simulink model "adcs_guidance"  (R2024b)
settings: Solver=VariableStepAuto  StartTime=0.0  StopTime=10.0  RelTol=1e-3
undefined symbols (not defined in the file): omega_thresh_high, omega_thresh_low
settings Model: DataDictionary=adcs_params.sldd  Creator=natha  LastModifiedBy=natha

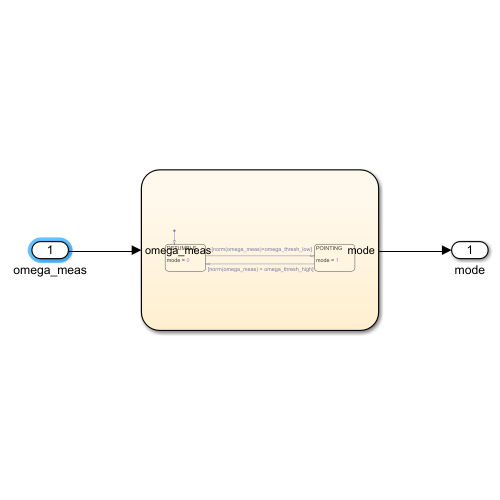
[thumbnail: Simulink's stored preview of the top-level diagram]
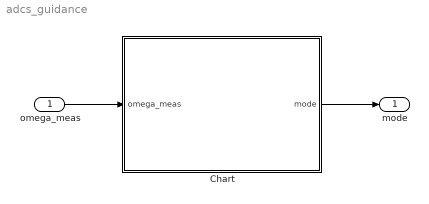
== system adcs_guidance ==
  omega_meas : Inport  PortDimensions=3
  Chart : Stateflow chart  TreatAsAtomicUnit=on
  mode : Outport
  wires:
  omega_meas/1 -> Chart/1(omega_meas)
  Chart/1(mode) -> mode/1

== stateflow chart adcs_guidance/Chart ==
  state DETUMBLE
    mode = 0
  state POINTING
    mode = 1
  (default) -> DETUMBLE
  DETUMBLE -> POINTING : [norm(omega_meas)<omega_thresh_low]
  POINTING -> DETUMBLE : [norm(omega_meas) > omega_thresh_high]
  data: mode output; omega_thresh_low parameter double; omega_thresh_high parameter double; omega_meas input size=3
